simulink model "Microgrid_transition_model_FORFIG"  (R2020a)
settings: Solver=VariableStepAuto  StartTime=0.0  StopTime=16  MaxStep=1e-4  RelTol=1e-3
PreLoadFcn:
  | %run('FC_microgrid_param.m')
  | %load('gen_grid_init.mat')
InitFcn:
  | %load myisoModel_init;
  | run('FC_microgrid_param.m')
  | tic
  | run('CARTinitFcn.m')
  | %caseNo = 2;
  | 
  | %if (caseNo == 1)
  | %set_param(['Isolated_grid_paper_model_022521/SignalGen'], 'ActiveScenario', 'PStep222kW');
  | %else
  | %set_param(['Isolated_grid_paper_model_022521/SignalGen'], 'ActiveScenario', 'QStep222kVAr');
  | 
  | %end;
StopFcn:
  | toc
undefined symbols (not defined in the file): breakpoints1, breakpoints2, cp_table_data, ctrl, D1, Delta, DiscIntNeverNeededParam, DT, FC_BESS, find_system, gcbh, libFC_BESS, LowerLimit, magnitude, oversize, pq_ts, sps_rtmsupport, timer, ts, Ts, Ts_APC, Ts_Control, Ts_Power, UpperLimit
libraries: powerlib x141, powerlib_meascontrol x104, simulink x73, powerlib_extras x60, simulink_extras x16, eePowerMeasurement x9, pi_ctrl x8, sps_avr x7, spsDieselMotorModel x3, SignalEditorBlockLib x2, libLgBattery x1, libFC_PV x1
(part 11 of 14)

== system Microgrid_transition_model_FORFIG/FC_BESS/SMAInverter/85_SMAControl/InvControl/CB_Meas2 ==
  Bus Creator : BusCreator  Inputs=9
  Bus Selector1 : BusSelector  OutputSignals=vabc_line,iabc
  Bus Selector2 : BusSelector  OutputSignals=vabc_line
  Bus Selector3 : BusSelector  OutputSignals=ejwt
  Bus Selector4 : BusSelector  OutputSignals=iabc
  Bus Selector5 : BusSelector  OutputSignals=ejwt
  Bus Selector6 : BusSelector  OutputSignals=vabc_inv
  Bus Selector7 : BusSelector  OutputSignals=ejwt
  Filter : Subsystem
  Filter1 : Subsystem
  InvMeas : Scope  NumInputPorts=7
  Math Function : Math  Operator=square  SignedPower=on  SaturateOnIntegerOverflow=on
  Math Function1 : Math  Operator=square  SignedPower=on  SaturateOnIntegerOverflow=on
  PQ_Calculator : Subsystem
  Sqrt : Sqrt  SaturateOnIntegerOverflow=on
  Sqrt1 : Sqrt  SaturateOnIntegerOverflow=on
  Sum of Elements : Sum  Inputs=+
  Sum of Elements1 : Sum  Inputs=+
  Unit Delay : UnitDelay  SampleTime=-1  HasFrameUpgradeWarning=on
  Unit Delay1 : UnitDelay  SampleTime=-1  HasFrameUpgradeWarning=on
  Unit Delay2 : UnitDelay  SampleTime=-1  HasFrameUpgradeWarning=on
  abc_to_dq0 Transformation : powerlib_extras/Measurements/abc_to_dq0 Transformation
      settings: SourceProductBaseCode=PS
  abc_to_dq0 Transformation1 : powerlib_extras/Measurements/abc_to_dq0 Transformation
      settings: SourceProductBaseCode=PS
  abc_to_dq0 Transformation2 : powerlib_extras/Measurements/abc_to_dq0 Transformation
      settings: SourceProductBaseCode=PS
  tag scope: cb_meas=scoped
  wires:
  PQ_Calculator/2(Q - kVAR) -> Bus Creator/2, InvMeas/6  "q"
  Filter/1(Out1) -> Bus Creator/4, InvMeas/2, Math Function/1
  Filter1/1(Out1) -> Bus Creator/7, InvMeas/4, Math Function1/1
  abc_to_dq0 Transformation1/1 -> Bus Creator/6, InvMeas/3, Filter1/1(In1)  "idq0"
  abc_to_dq0 Transformation/1 -> Bus Creator/3, InvMeas/1, Filter/1(In1)  "vdq0"
  PQ_Calculator/1(P - kW) -> InvMeas/5, Bus Creator/1  "p"
  Unit Delay1/1 -> abc_to_dq0 Transformation1/2
  Unit Delay/1 -> abc_to_dq0 Transformation/2
  [cb_pu] -> Bus Selector4/1
  Sqrt1/1 -> Bus Creator/8  "irms"
  Sum of Elements1/1 -> Sqrt1/1
  Math Function1/1 -> Sum of Elements1/1
  Bus Selector5/1 -> Unit Delay1/1  "<ejwt>"
  [pll] -> Bus Selector5/1
  Bus Selector4/1 -> abc_to_dq0 Transformation1/1  "<iabc>"
  [cb_pu] -> Bus Selector2/1
  Sqrt/1 -> Bus Creator/5  "vrms"
  Sum of Elements/1 -> Sqrt/1
  Math Function/1 -> Sum of Elements/1
  Bus Selector3/1 -> Unit Delay/1  "<ejwt>"
  [pll] -> Bus Selector3/1
  Bus Selector2/1 -> abc_to_dq0 Transformation/1  "<vabc_line>"
  Bus Selector1/2 -> PQ_Calculator/2(Iabc)  "<iabc>"
  Bus Creator/1 -> [cb_meas]
  Bus Selector1/1 -> PQ_Calculator/1(Vabc)  "<vabc_line>"
  [cb_pu] -> Bus Selector1/1
  Bus Selector7/1 -> Unit Delay2/1  "<ejwt>"
  [pll] -> Bus Selector7/1
  [cb_pu] -> Bus Selector6/1
  Bus Selector6/1 -> abc_to_dq0 Transformation2/1  "<vabc_inv>"
  Unit Delay2/1 -> abc_to_dq0 Transformation2/2
  abc_to_dq0 Transformation2/1 -> InvMeas/7, Bus Creator/9  "vdq0_inv"

== system Microgrid_transition_model_FORFIG/FC_BESS/SMAInverter/85_SMAControl/InvControl/CB_pu ==
  Bus Creator : BusCreator  Inputs=3
  Bus Selector1 : BusSelector  OutputSignals=Uabc,Uabc_inv
  Bus Selector2 : BusSelector  OutputSignals=Iabc
  Gain : Gain  Gain=1/Unom/sqrt(2)
  Gain1 : Gain  Gain=1/Inom/sqrt(2)
  Gain2 : Gain  Gain=1/Unom/sqrt(2)
  tag scope: cb_pu=scoped
  wires:
  Gain1/1 -> Bus Creator/3  "iabc"
  Bus Selector2/1 -> Gain1/1  "<Iabc>"
  [inputs] -> Bus Selector2/1
  [inputs] -> Bus Selector1/1
  Bus Selector1/1 -> Gain/1  "<Uabc>"
  Gain/1 -> Bus Creator/1  "vabc_line"
  Bus Creator/1 -> [cb_pu]
  Bus Selector1/2 -> Gain2/1  "<Uabc_inv>"
  Gain2/1 -> Bus Creator/2  "vabc_inv"

== system Microgrid_transition_model_FORFIG/FC_BESS/SMAInverter/85_SMAControl/InvControl/CS_controller ==
  Bias : Bias  Bias=(1.5*Ts)*60*2*pi
  Bus Creator : BusCreator  Inputs=3
  Bus Selector10 : BusSelector  OutputSignals=cb_status,Control_Word.GF_mode
  Bus Selector2 : BusSelector  OutputSignals=udq
  Bus Selector3 : BusSelector  OutputSignals=udq
  Bus Selector5 : BusSelector  OutputSignals=wt
  Constant : Constant  Value=0
  Constant2 : Constant  Value=1.3
  Gain1 : Gain  Gain=-1
  Gain2 : Gain  Gain=Unom*sqrt(2)
  Logical Operator : Logic  AllPortsSameDT=off  OutDataTypeStr=boolean
  Logical Operator1 : Logic  Operator=NOT  AllPortsSameDT=off  OutDataTypeStr=boolean
  Mux1 : Mux  Inputs=2
  Mux3 : Mux  Inputs=2
  Saturation Dynamic : simulink/Discontinuities/Saturation Dynamic  OutMin=[]  OutMax=[]  OutDataTypeStr=Inherit: Same as second input  OutDataType=fixdt(1, 16)  OutScaling=2^-10  DoSatur=off
  Scope : Scope  NumInputPorts=2
  Switch : Switch  Criteria=u2 > Threshold
  Trigonometric Function2 : Trigonometry
  Trigonometric Function3 : Trigonometry  Operator=cos
  dq0_to_abc Transformation : powerlib_extras/Measurements/dq0_to_abc Transformation
      settings: SourceProductBaseCode=PS
  tag scope: inverter=scoped
  wires:
  [use_csi] -> Bus Creator/2  "use_csi"
  Bus Selector3/1 -> Switch/1  "<udq>"
  [I_Ctrl] -> Bus Selector3/1
  Logical Operator/1 -> Switch/2, Scope/1, [use_csi]
  [V_Ctrl] -> Bus Selector2/1
  Bus Selector2/1 -> Switch/3  "<udq>"
  [inputs] -> Bus Selector10/1
  Bus Selector10/2 -> Logical Operator1/1  "<GF_mode>"
  Logical Operator1/1 -> Logical Operator/2
  Bus Selector10/1 -> Logical Operator/1  "<cb_status>"
  Switch/1 -> Mux1/1, Bus Creator/3, Scope/2  "vdq"
  Mux1/1 -> dq0_to_abc Transformation/1
  Constant/1 -> Mux1/2
  Mux3/1 -> [ejwt]
  Trigonometric Function2/1 -> Mux3/1
  Trigonometric Function3/1 -> Mux3/2
  Bias/1 -> Trigonometric Function3/1, Trigonometric Function2/1
  Gain2/1 -> Bus Creator/1  "Uabc_ref"
  Constant2/1 -> Saturation Dynamic/1, Gain1/1
  Gain1/1 -> Saturation Dynamic/3
  Bus Creator/1 -> [inverter]
  dq0_to_abc Transformation/1 -> Saturation Dynamic/2
  [ejwt] -> dq0_to_abc Transformation/2
  Saturation Dynamic/1 -> Gain2/1  "uabc_ref"
  [pll] -> Bus Selector5/1
  Bus Selector5/1 -> Bias/1  "<wt>"

== system Microgrid_transition_model_FORFIG/FC_BESS/SMAInverter/85_SMAControl/InvControl/Droop ==
  Bus Selector1 : BusSelector  OutputSignals=vrms
  Bus Selector2 : BusSelector  OutputSignals=freq
  Bus Selector3 : BusSelector  OutputSignals=p,q,idq0
  Bus Selector9 : BusSelector  OutputSignals=fref,vref,pref,qref  OutputAsBus=on
  Constant : Constant  Value=[0 0]
  Demux : Demux
  Demux1 : Demux
  Droop : Subsystem
  ExtractCoefs : Subsystem
  Gain : Gain  Gain=[1 -1]
  Mux : Mux  Inputs=3
  Mux1 : Mux  Inputs=2
  Mux2 : Mux  Inputs=2
  Scope : Scope  NumInputPorts=4
  Scope1 : Scope  NumInputPorts=4
  Selector1 : Selector  InputPortWidth=4  IndexOptions=Index vector (dialog)  Indices=[1 2]  OutputSizes=1
  Selector2 : Selector  InputPortWidth=3  IndexOptions=Index vector (dialog)  Indices=[1 2]  OutputSizes=1
  Sum1 : Sum  Inputs=-+|
  Sum2 : Sum  Inputs=++|
  Terminator : Terminator
  tag scope: droop=scoped
  wires:
  Demux1/4 -> Scope1/4
  Demux1/1 -> Scope1/1
  Demux1/2 -> Scope1/2
  Demux1/3 -> Scope1/3
  Sum2/1 -> [droop], Demux1/1  "fvpq_meas"
  Gain/1 -> Mux/3
  Selector2/1 -> Gain/1
  Mux2/1 -> Terminator/1
  Bus Selector3/3 -> Selector2/1  "<idq0>"
  Bus Selector3/2 -> Mux2/2  "<q>"
  Bus Selector3/1 -> Mux2/1  "<p>"
  [cb_meas] -> Bus Selector3/1
  Demux/4 -> Scope/4
  Demux/3 -> Scope/3
  Demux/2 -> Scope/2
  Demux/1 -> Scope/1
  Bus Selector2/1 -> Mux/1  "<freq>"
  Bus Selector1/1 -> Mux/2  "<vrms>"
  [pll] -> Bus Selector2/1
  ExtractCoefs/1(Out1) -> Droop/2(droop)
  [inputs] -> ExtractCoefs/1(In1)
  Mux/1 -> Demux/1, Sum1/1  "fvpq_meas"
  [cb_meas] -> Bus Selector1/1
  Bus Selector9/1 -> Selector1/1, Sum2/2
  [inputs] -> Bus Selector9/1
  Droop/1(dFvpq_out) -> Sum2/1
  Sum1/1 -> Droop/1(dfvpq)
  Selector1/1 -> Mux1/1
  Mux1/1 -> Sum1/2
  Constant/1 -> Mux1/2

== system Microgrid_transition_model_FORFIG/FC_BESS/SMAInverter/85_SMAControl/InvControl/PLL ==
  note: Rising and falling edge debounce
  Aligned : simulink/Logic and Bit Operations/Interval Test  IntervalClosedRight=on  uplimit=0.05  IntervalClosedLeft=on  lowlimit=-0.05  OutDataTypeStr=boolean
  Aligned1 : simulink/Logic and Bit Operations/Interval Test  IntervalClosedRight=on  uplimit=1.25  IntervalClosedLeft=on  lowlimit=0.05  OutDataTypeStr=boolean
  Bus Creator : BusCreator  Inputs=5
  Bus Selector10 : BusSelector  OutputSignals=Control_Word.GF_mode
  Bus Selector2 : BusSelector  OutputSignals=vabc_line
  Bus Selector8 : BusSelector  OutputSignals=cb_status
  Constant : Constant  Value=0
  Data Type Conversion : DataTypeConversion
  DebounceAlternative : Subsystem  mask{Tdb_off=0.05, Tdb_on=0.2, Tdb_sample=Ts}
      mask prompts: Tdb_off "Debounce Time When OFF"; Tdb_on "Debounce Time When On"; Tdb_sample "Sample Time"
      mask Display: disp(['Debouncing unit\nTdb when off is ' num2str(Tdb_off) '\nTdb when on is ' num2str(Tdb_on)]);
  Display : Display
  Gain : Gain  Gain=1/60
  Gain1 : Gain  Gain=2*pi*60  SaturateOnIntegerOverflow=on  OutDataTypeStr=Inherit: Same as input  ParamDataTypeStr=Inherit: Same as input
  Logical Operator1 : Logic  AllPortsSameDT=off  OutDataTypeStr=boolean
  Logical Operator2 : Logic  AllPortsSameDT=off  OutDataTypeStr=boolean
  Logical Operator3 : Logic  AllPortsSameDT=off  OutDataTypeStr=boolean
  Logical Operator{4..6,8} (4 alike) : Logic  Operator=NOT  AllPortsSameDT=off  OutDataTypeStr=boolean
  Logical Operator7 : Logic  Operator=OR  AllPortsSameDT=off  OutDataTypeStr=boolean
  Mux3 : Mux  Inputs=2
  PLL (3ph)1 : Subsystem  DialogController=POWERSYS.PowerSysDialog  LoadFcn=sps_rtmsupport('LoadFcn', gcbh);  StartFcn=sps_rtmsupport('StartFcn', gcbh);  StopFcn=sps_rtmsupport('StopFcn', gcbh);  mask(PLL (3ph)){Flim=[55 66], Par_Init=[90, 60], ParK=[pll_kp, pll_ki, 1], TcD=Ts, MaxRateChangeFreq=12, FilterCutOffFreq=25, Ts=Ts, AGC=off}
      mask prompts: Flim "Minimum frequency (Hz):"; Par_Init "Initial inputs [ Phase (degrees), Frequency (Hz) ]:"; ParK "Regulator gains [ Kp, Ki, Kd ]:"; TcD "Time constant for derivative action (s):"; MaxRateChangeFreq "Maximum rate of change of frequency (Hz/s):"; FilterCutOffFreq "Filter cut-off frequency for frequency measurement (Hz):"; Ts "Sample time:"; AGC "Enable automatic gain control"
      mask help:
      | This Phase Locked Loop (PLL) system can be used  to synchronize on a set of variable frequency, three-phase sinusoidal signals. If the Automatic Gain Control is enabled, the input (phase error) of the PLL regulator is scaled according to the input signals magnitude.
      |
      | For optimal performance, set regulator gains [ Kp Ki  Kd ] = [ 180  3200  1 ] and check the Enable Automatic Gain Control parameter.
      |
      | Input : Vector containing the normalized three-phase signals [Va Vb Vc]
      | Output 1:  Measured frequency (Hz) = w/(2pi)
      | Output 2:  Ramp w.t varying between  0 and 2*pi, synchronized on zero crossings of the fundamental (positive-sequence) of phase A.
      mask init:
      | %block=gcb;
      | %[WantBlockChoice,Ts,sps] = powericon('PLL3phInit',block,Fmin,Par_Init,ParK,TcD, MaxRateChangeFreq, FilterCutOffFreq, AGC,Ts);
      | %powericon('SetInternalModels','set',block,WantBlockChoice);
      settings: CopyFcn=sps_rtmsupport('CopyFcn', gcbh);  DeleteFcn=sps_rtmsupport('DeleteFcn', gcbh);  UndoDeleteFcn=sps_rtmsupport('UndoDeleteFcn', gcbh);  ModelCloseFcn=sps_rtmsupport('ModelCloseFcn', gcbh);  PreSaveFcn=sps_rtmsupport('PreSaveFcn', gcbh);  PostSaveFcn=sps_rtmsupport('PostSaveFcn', gcbh);  NameChangeFcn=sps_rtmsupport('NameChangeFcn', gcbh);  PreCopyFcn=sps_rtmsupport('PreCopyFcn', gcbh);  CloseFcn=sps_rtmsupport('CloseFcn', gcbh);  PreDeleteFcn=sps_rtmsupport('PreDeleteFcn', gcbh);
      settings: OpenFcn=|
      | power_openblockproxy();
      | sps_rtmsupport('OpenFcn', gcbh, [8]);
      mask Help: helpview(psbhelp);
  Scope : Scope  NumInputPorts=5
  Selector1 : Selector  InputPortWidth=3  IndexOptions=Index vector (dialog)  Indices=1  OutputSizes=1
  Selector2 : Selector  InputPortWidth=3  IndexOptions=Index vector (dialog)  Indices=2  OutputSizes=1
  Selector3 : Selector  InputPortWidth=4  IndexOptions=Index vector (dialog)  Indices=[1]  OutputSizes=1
  Switch : Switch  Criteria=u2 > Threshold
  Terminator : Terminator
  Trigonometric Function2 : Trigonometry
  Trigonometric Function3 : Trigonometry  Operator=cos
  VCO : Subsystem
  tag scope: pll=scoped
  wires:
  Switch/1 -> Bus Creator/3, Scope/5, Trigonometric Function2/1, Trigonometric Function3/1  "wt"
  PLL (3ph)1/3(dq0) -> Selector2/1, Selector1/1
  Logical Operator7/1 -> Scope/1, [use_pll]  "use_pll"
  Logical Operator3/1 -> Logical Operator7/2
  Logical Operator5/1 -> Logical Operator3/2
  Logical Operator4/1 -> Logical Operator3/1
  Bus Selector10/1 -> Logical Operator5/1  "<GF_mode>"
  Logical Operator1/1 -> Logical Operator7/1
  [lock] -> Logical Operator1/2
  [cb_open] -> Logical Operator1/1, Scope/4, Logical Operator4/1  "cb_open"
  Bus Selector8/1 -> Logical Operator8/1  "<cb_status>"
  Logical Operator8/1 -> Display/1, [cb_open]
  [inputs] -> Bus Selector8/1
  [inputs] -> Bus Selector10/1
  Trigonometric Function3/1 -> Mux3/2
  Trigonometric Function2/1 -> Mux3/1
  Mux3/1 -> Bus Creator/4  "ejwt"
  Logical Operator6/1 -> Switch/2
  [use_pll] -> VCO/2(rst), Logical Operator6/1
  VCO/1(theta) -> Switch/1
  Gain1/1 -> VCO/1(w)
  [ref_lim] -> Selector3/1
  Selector3/1 -> Scope/3, Gain1/1
  Gain/1 -> Bus Creator/1  "freq"
  PLL (3ph)1/2(wt) -> VCO/3(init), Switch/3  "wt"
  Bus Selector2/1 -> PLL (3ph)1/1(abc)  "<vabc_line>"
  [cb_pu] -> Bus Selector2/1
  Data Type Conversion/1 -> DebounceAlternative/1(In)
  Constant/1 -> DebounceAlternative/2(Rst)
  DebounceAlternative/2(IntOut) -> Terminator/1
  Logical Operator2/1 -> Data Type Conversion/1
  Selector2/1 -> Aligned/1
  Selector1/1 -> Aligned1/1
  Aligned1/1 -> Logical Operator2/2
  Aligned/1 -> Logical Operator2/1
  DebounceAlternative/1(Out) -> Scope/2, [lock], Bus Creator/5  "lock"
  PLL (3ph)1/1(Freq) -> Gain/1, Bus Creator/2  "Freq"
  Bus Creator/1 -> [pll]

== system Microgrid_transition_model_FORFIG/FC_BESS/SMAInverter/85_SMAControl/InvControl/Ref_Limiting ==
  Constant : Constant
  Constant1 : Constant  Value=-1
  Demux : Demux
  RefLimiting : Subsystem
  Scope : Scope  NumInputPorts=4
  tag scope: ref_lim=scoped
  wires:
  Demux/4 -> Scope/4
  Demux/3 -> Scope/3
  Demux/2 -> Scope/2
  Demux/1 -> Scope/1
  [droop] -> RefLimiting/1(fvpq_in)
  Constant/1 -> RefLimiting/2(p_max)
  Constant1/1 -> RefLimiting/3(p_min)
  RefLimiting/1(fvpq_out) -> Demux/1, [ref_lim]  "FVPQ"

== system Microgrid_transition_model_FORFIG/MODEL STABILIZER/AllStringInverters/Stab_control/InvControl/40_V_Control ==
  Add1 : Sum  Inputs=+-
  Bus Creator : BusCreator  Inputs=1
  Bus Selector1 : BusSelector  OutputSignals=vdq0_inv  OutputAsBus=on
  Bus Selector8 : BusSelector  OutputSignals=use_csi,vdq
  Constant1 : Constant  Value=double(0)
  Constant2 : Constant  Value=10  OutDataTypeStr=double
  Demux : Demux  Outputs=2
  Demux1 : Demux  Outputs=2
  Logical Operator : Logic  Operator=NOT  Inputs=1  AllPortsSameDT=off  OutDataTypeStr=boolean
  Manual Switch2 : ManualSwitch  CurrentSetting=0
  Mux2 : Mux  Inputs=2
  Mux8 : Mux  Inputs=2
  PI_controller_with_reset : pi_ctrl/PI_controller_with_reset  Kp=0.0005  Ti=0.02  Ts=Ts  Iup=1.5  Idown=0  PIup=1.5  PIdown=0
  PI_controller_with_reset1 : pi_ctrl/PI_controller_with_reset  Kp=0.0005  Ti=0.02  Ts=Ts  Iup=1.5  Idown=-1  PIup=1.5  PIdown=-1
  Scope : Scope  NumInputPorts=4
  Selector : Selector  InputPortWidth=4  IndexOptions=Index vector (dialog)  Indices=2  OutputSizes=1
  Selector2 : Selector  InputPortWidth=3  IndexOptions=Index vector (dialog)  Indices=[1 2]  OutputSizes=1
  Subsystem : Subsystem  mask{Ts=Ts}
      mask prompts: Ts "Sampling time"
  Unit Delay : UnitDelay  SampleTime=-1  HasFrameUpgradeWarning=on
  Unit Delay1 : UnitDelay  InitialCondition=[0 0]  SampleTime=-1  HasFrameUpgradeWarning=on
  tag scope: V_Ctrl=scoped
  wires:
  [ref_lim] -> Selector/1
  Bus Creator/1 -> [V_Ctrl]
  Mux8/1 -> Scope/3, Unit Delay/1, Bus Creator/1  "udq"
  [cb_meas] -> Bus Selector1/1
  Bus Selector1/1 -> Selector2/1
  PI_controller_with_reset/1 -> Mux8/1, Scope/4
  Demux1/1 -> PI_controller_with_reset/1
  Demux1/2 -> PI_controller_with_reset1/1
  Add1/1 -> Demux1/1
  Subsystem/1(out) -> Add1/1, Scope/1
  Manual Switch2/1 -> Add1/2, Scope/2
  Selector/1 -> Mux2/1
  Constant1/1 -> Mux2/2
  [inverter] -> Bus Selector8/1
  PI_controller_with_reset1/1 -> Mux8/2
  Logical Operator/1 -> PI_controller_with_reset1/2, PI_controller_with_reset/2
  Bus Selector8/2 -> Unit Delay1/1  "<vdq>"
  Demux/1 -> PI_controller_with_reset/3
  Demux/2 -> PI_controller_with_reset1/3
  Selector2/1 -> Manual Switch2/2
  Unit Delay/1 -> Manual Switch2/1
  Bus Selector8/1 -> Subsystem/2(rst), Logical Operator/1  "<use_csi>"
  Mux2/1 -> Subsystem/1(in)
  Constant2/1 -> Subsystem/4(rate)
  Unit Delay1/1 -> Subsystem/3(init), Demux/1

== system Microgrid_transition_model_FORFIG/MODEL STABILIZER/AllStringInverters/Stab_control/InvControl/50_I_Control ==
  Add1 : Sum  Inputs=+-
  Bus Creator : BusCreator  Inputs=1
  Bus Selector1 : BusSelector  OutputSignals=idq0  OutputAsBus=on
  Bus Selector2 : BusSelector  OutputSignals=use_csi,vdq
  Bus Selector3 : BusSelector  OutputSignals=vdq0_inv  OutputAsBus=on
  Constant : Constant  Value=10  OutDataTypeStr=double
  Demux : Demux  Outputs=2
  Demux1 : Demux  Outputs=2
  Filter : Subsystem
  Filter1 : Subsystem
  Gain : Gain
  Gain1 : Gain
  Logical Operator : Logic  Operator=NOT  Inputs=1  AllPortsSameDT=off  OutDataTypeStr=boolean
  Mux8 : Mux  Inputs=2
  PI_controller_with_reset : pi_ctrl/PI_controller_with_reset  Kp=cc_kp  Ti=cc_Ti  Ts=Ts  Iup=1.5  Idown=-0.5  PIup=1.5  PIdown=-0.5
  PI_controller_with_reset1 : pi_ctrl/PI_controller_with_reset  Kp=cc_kp  Ti=0.6e-3*100  Ts=Ts  Iup=1  Idown=-1  PIup=1  PIdown=-1
  Scope : Scope  NumInputPorts=3
  Selector : Selector  InputPortWidth=4  IndexOptions=Index vector (dialog)  Indices=[3 4]  OutputSizes=1
  Selector1 : Selector  InputPortWidth=3  IndexOptions=Index vector (dialog)  Indices=[1 2]  OutputSizes=1
  Selector2 : Selector  InputPortWidth=3  IndexOptions=Index vector (dialog)  Indices=[1 2]  OutputSizes=1
  Subsystem : Subsystem  mask{Ts=Ts}
      mask prompts: Ts "Sampling time"
  Sum : Sum  Inputs=|++
  Sum1 : Sum  Inputs=|+-
  Unit Delay : UnitDelay  SampleTime=-1  HasFrameUpgradeWarning=on
  tag scope: I_Ctrl=scoped
  wires:
  Gain1/1 -> Sum/2
  Gain/1 -> Sum1/2
  Filter1/1(Out1) -> Gain/1, Gain1/1
  Selector1/1 -> Filter1/1(In1)
  Bus Selector3/1 -> Selector1/1
  [cb_meas] -> Bus Selector3/1
  Sum1/1 -> Demux/1  "udq"
  Mux8/1 -> Scope/2, Sum/1  "udq"
  Filter/1(Out1) -> Add1/2
  Selector2/1 -> Filter/1(In1), Subsystem/3(init)
  Subsystem/1(out) -> Add1/1
  Add1/1 -> Demux1/1
  Demux1/2 -> PI_controller_with_reset1/1
  Demux1/1 -> PI_controller_with_reset/1
  PI_controller_with_reset/1 -> Mux8/1
  Bus Selector1/1 -> Selector2/1
  [cb_meas] -> Bus Selector1/1
  Sum/1 -> Bus Creator/1, Scope/3  "udq"
  Bus Creator/1 -> [I_Ctrl]
  [ref_lim] -> Selector/1
  [inverter] -> Bus Selector2/1
  Bus Selector2/1 -> PI_controller_with_reset/2, Scope/1, PI_controller_with_reset1/2, Logical Operator/1  "<use_csi>"
  Bus Selector2/2 -> Unit Delay/1  "<vdq>"
  Demux/1 -> PI_controller_with_reset/3
  Demux/2 -> PI_controller_with_reset1/3
  Selector/1 -> Subsystem/1(in)
  Constant/1 -> Subsystem/4(rate)
  Logical Operator/1 -> Subsystem/2(rst)
  Unit Delay/1 -> Sum1/1
  PI_controller_with_reset1/1 -> Mux8/2

== system Microgrid_transition_model_FORFIG/MODEL STABILIZER/AllStringInverters/Stab_control/InvControl/CB_Meas2 ==
  Bus Creator : BusCreator  Inputs=9
  Bus Selector1 : BusSelector  OutputSignals=vabc_line,iabc
  Bus Selector2 : BusSelector  OutputSignals=vabc_line
  Bus Selector3 : BusSelector  OutputSignals=ejwt
  Bus Selector4 : BusSelector  OutputSignals=iabc
  Bus Selector5 : BusSelector  OutputSignals=ejwt
  Bus Selector6 : BusSelector  OutputSignals=vabc_inv
  Bus Selector7 : BusSelector  OutputSignals=ejwt
  Filter : Subsystem
  Filter1 : Subsystem
  Math Function : Math  Operator=square  SignedPower=on  SaturateOnIntegerOverflow=on
  Math Function1 : Math  Operator=square  SignedPower=on  SaturateOnIntegerOverflow=on
  PQ_Calculator : Subsystem
  Sqrt : Sqrt  SaturateOnIntegerOverflow=on
  Sqrt1 : Sqrt  SaturateOnIntegerOverflow=on
  Sum of Elements : Sum  Inputs=+
  Sum of Elements1 : Sum  Inputs=+
  Unit Delay : UnitDelay  SampleTime=-1  HasFrameUpgradeWarning=on
  Unit Delay1 : UnitDelay  SampleTime=-1  HasFrameUpgradeWarning=on
  Unit Delay2 : UnitDelay  SampleTime=-1  HasFrameUpgradeWarning=on
  abc_to_dq0 Transformation : powerlib_extras/Measurements/abc_to_dq0 Transformation
      settings: SourceProductBaseCode=PS
  abc_to_dq0 Transformation1 : powerlib_extras/Measurements/abc_to_dq0 Transformation
      settings: SourceProductBaseCode=PS
  abc_to_dq0 Transformation2 : powerlib_extras/Measurements/abc_to_dq0 Transformation
      settings: SourceProductBaseCode=PS
  tag scope: cb_meas=scoped
  wires:
  abc_to_dq0 Transformation2/1 -> Bus Creator/9  "vdq0_inv"
  Unit Delay2/1 -> abc_to_dq0 Transformation2/2
  Bus Selector6/1 -> abc_to_dq0 Transformation2/1  "<vabc_inv>"
  [cb_pu] -> Bus Selector6/1
  [pll] -> Bus Selector7/1
  Bus Selector7/1 -> Unit Delay2/1  "<ejwt>"
  [cb_pu] -> Bus Selector1/1
  Bus Selector1/1 -> PQ_Calculator/1(Vabc)  "<vabc_line>"
  Bus Creator/1 -> [cb_meas]
  Bus Selector1/2 -> PQ_Calculator/2(Iabc)  "<iabc>"
  Bus Selector2/1 -> abc_to_dq0 Transformation/1  "<vabc_line>"
  [pll] -> Bus Selector3/1
  Bus Selector3/1 -> Unit Delay/1  "<ejwt>"
  Math Function/1 -> Sum of Elements/1
  Sum of Elements/1 -> Sqrt/1
  Sqrt/1 -> Bus Creator/5  "vrms"
  [cb_pu] -> Bus Selector2/1
  Bus Selector4/1 -> abc_to_dq0 Transformation1/1  "<iabc>"
  [pll] -> Bus Selector5/1
  Bus Selector5/1 -> Unit Delay1/1  "<ejwt>"
  Math Function1/1 -> Sum of Elements1/1
  Sum of Elements1/1 -> Sqrt1/1
  Sqrt1/1 -> Bus Creator/8  "irms"
  [cb_pu] -> Bus Selector4/1
  Unit Delay/1 -> abc_to_dq0 Transformation/2
  Unit Delay1/1 -> abc_to_dq0 Transformation1/2
  PQ_Calculator/1(P - kW) -> Bus Creator/1  "p"
  abc_to_dq0 Transformation/1 -> Filter/1(In1), Bus Creator/3  "vdq0"
  abc_to_dq0 Transformation1/1 -> Filter1/1(In1), Bus Creator/6  "idq0"
  Filter1/1(Out1) -> Math Function1/1, Bus Creator/7
  Filter/1(Out1) -> Math Function/1, Bus Creator/4
  PQ_Calculator/2(Q - kVAR) -> Bus Creator/2  "q"

== system Microgrid_transition_model_FORFIG/MODEL STABILIZER/AllStringInverters/Stab_control/InvControl/CB_pu ==
  Bus Creator : BusCreator  Inputs=3
  Bus Selector1 : BusSelector  OutputSignals=Uabc,Uabc_inv
  Bus Selector2 : BusSelector  OutputSignals=Iabc
  Gain : Gain  Gain=1/Unom/sqrt(2)
  Gain1 : Gain  Gain=1/Inom/sqrt(2)
  Gain2 : Gain  Gain=1/Unom/sqrt(2)
  tag scope: cb_pu=scoped
  wires:
  Gain2/1 -> Bus Creator/2  "vabc_inv"
  Bus Selector1/2 -> Gain2/1  "<Uabc_inv>"
  Bus Creator/1 -> [cb_pu]
  Gain/1 -> Bus Creator/1  "vabc_line"
  Bus Selector1/1 -> Gain/1  "<Uabc>"
  [inputs] -> Bus Selector1/1
  [inputs] -> Bus Selector2/1
  Bus Selector2/1 -> Gain1/1  "<Iabc>"
  Gain1/1 -> Bus Creator/3  "iabc"

== system Microgrid_transition_model_FORFIG/MODEL STABILIZER/AllStringInverters/Stab_control/InvControl/CS_controller ==
  Bias : Bias  Bias=(1.5*Ts)*60*2*pi
  Bus Creator : BusCreator  Inputs=3
  Bus Selector10 : BusSelector  OutputSignals=cb_status,Control_Word.GF_mode
  Bus Selector2 : BusSelector  OutputSignals=udq
  Bus Selector3 : BusSelector  OutputSignals=udq
  Bus Selector5 : BusSelector  OutputSignals=wt
  Constant : Constant  Value=0
  Constant2 : Constant  Value=1.3
  Gain1 : Gain  Gain=-1
  Gain2 : Gain  Gain=Unom*sqrt(2)
  Logical Operator : Logic  AllPortsSameDT=off  OutDataTypeStr=boolean
  Logical Operator1 : Logic  Operator=NOT  AllPortsSameDT=off  OutDataTypeStr=boolean
  Mux1 : Mux  Inputs=2
  Mux3 : Mux  Inputs=2
  Saturation Dynamic : simulink/Discontinuities/Saturation Dynamic  OutMin=[]  OutMax=[]  OutDataTypeStr=Inherit: Same as second input  OutDataType=fixdt(1, 16)  OutScaling=2^-10  DoSatur=off
  Scope : Scope  NumInputPorts=2
  Switch : Switch  Criteria=u2 > Threshold
  Trigonometric Function2 : Trigonometry
  Trigonometric Function3 : Trigonometry  Operator=cos
  dq0_to_abc Transformation : powerlib_extras/Measurements/dq0_to_abc Transformation
      settings: SourceProductBaseCode=PS
  tag scope: inverter=scoped
  wires:
  Bus Selector5/1 -> Bias/1  "<wt>"
  [pll] -> Bus Selector5/1
  Saturation Dynamic/1 -> Gain2/1  "uabc_ref"
  [ejwt] -> dq0_to_abc Transformation/2
  dq0_to_abc Transformation/1 -> Saturation Dynamic/2
  Bus Creator/1 -> [inverter]
  Gain1/1 -> Saturation Dynamic/3
  Constant2/1 -> Gain1/1, Saturation Dynamic/1
  Gain2/1 -> Bus Creator/1  "Uabc_ref"
  Bias/1 -> Trigonometric Function2/1, Trigonometric Function3/1
  Trigonometric Function3/1 -> Mux3/2
  Trigonometric Function2/1 -> Mux3/1
  Mux3/1 -> [ejwt]
  Constant/1 -> Mux1/2
  Mux1/1 -> dq0_to_abc Transformation/1
  Switch/1 -> Scope/2, Bus Creator/3, Mux1/1  "vdq"
  Bus Selector10/1 -> Logical Operator/1  "<cb_status>"
  Logical Operator1/1 -> Logical Operator/2
  Bus Selector10/2 -> Logical Operator1/1  "<GF_mode>"
  [inputs] -> Bus Selector10/1
  Bus Selector2/1 -> Switch/3  "<udq>"
  [V_Ctrl] -> Bus Selector2/1
  Logical Operator/1 -> [use_csi], Scope/1, Switch/2
  [I_Ctrl] -> Bus Selector3/1
  Bus Selector3/1 -> Switch/1  "<udq>"
  [use_csi] -> Bus Creator/2  "use_csi"

== system Microgrid_transition_model_FORFIG/MODEL STABILIZER/AllStringInverters/Stab_control/InvControl/Droop ==
  Bus Selector1 : BusSelector  OutputSignals=vrms
  Bus Selector2 : BusSelector  OutputSignals=freq
  Bus Selector3 : BusSelector  OutputSignals=p,q,idq0
  Bus Selector9 : BusSelector  OutputSignals=fref,vref,pref,qref  OutputAsBus=on
  Constant : Constant  Value=[0 0]
  Demux : Demux
  Demux1 : Demux
  Droop : Subsystem
  ExtractCoefs : Subsystem
  Gain : Gain  Gain=[1 -1]
  Mux : Mux  Inputs=3
  Mux1 : Mux  Inputs=2
  Mux2 : Mux  Inputs=2
  Scope : Scope  NumInputPorts=4
  Scope1 : Scope  NumInputPorts=4
  Selector1 : Selector  InputPortWidth=4  IndexOptions=Index vector (dialog)  Indices=[1 2]  OutputSizes=1
  Selector2 : Selector  InputPortWidth=3  IndexOptions=Index vector (dialog)  Indices=[1 2]  OutputSizes=1
  Sum1 : Sum  Inputs=-+|
  Sum2 : Sum  Inputs=++|
  Terminator : Terminator
  tag scope: droop=scoped
  wires:
  Constant/1 -> Mux1/2
  Mux1/1 -> Sum1/2
  Selector1/1 -> Mux1/1
  Sum1/1 -> Droop/1(dfvpq)
  Droop/1(dFvpq_out) -> Sum2/1
  [inputs] -> Bus Selector9/1
  Bus Selector9/1 -> Sum2/2, Selector1/1
  [cb_meas] -> Bus Selector1/1
  Mux/1 -> Sum1/1, Demux/1  "fvpq_meas"
  [inputs] -> ExtractCoefs/1(In1)
  ExtractCoefs/1(Out1) -> Droop/2(droop)
  [pll] -> Bus Selector2/1
  Bus Selector1/1 -> Mux/2  "<vrms>"
  Bus Selector2/1 -> Mux/1  "<freq>"
  Demux/1 -> Scope/1
  Demux/2 -> Scope/2
  Demux/3 -> Scope/3
  Demux/4 -> Scope/4
  [cb_meas] -> Bus Selector3/1
  Bus Selector3/1 -> Mux2/1  "<p>"
  Bus Selector3/2 -> Mux2/2  "<q>"
  Bus Selector3/3 -> Selector2/1  "<idq0>"
  Mux2/1 -> Terminator/1
  Selector2/1 -> Gain/1
  Gain/1 -> Mux/3
  Sum2/1 -> Demux1/1, [droop]  "fvpq_meas"
  Demux1/3 -> Scope1/3
  Demux1/2 -> Scope1/2
  Demux1/1 -> Scope1/1
  Demux1/4 -> Scope1/4

== system Microgrid_transition_model_FORFIG/MODEL STABILIZER/AllStringInverters/Stab_control/InvControl/PLL ==
  note: Rising and falling edge debounce
  Aligned : simulink/Logic and Bit Operations/Interval Test  IntervalClosedRight=on  uplimit=0.05  IntervalClosedLeft=on  lowlimit=-0.05  OutDataTypeStr=boolean
  Aligned1 : simulink/Logic and Bit Operations/Interval Test  IntervalClosedRight=on  uplimit=1.25  IntervalClosedLeft=on  lowlimit=0.05  OutDataTypeStr=boolean
  Bus Creator : BusCreator  Inputs=5
  Bus Selector10 : BusSelector  OutputSignals=Control_Word.GF_mode
  Bus Selector2 : BusSelector  OutputSignals=vabc_line
  Bus Selector8 : BusSelector  OutputSignals=cb_status
  Constant : Constant  Value=0
  Data Type Conversion : DataTypeConversion
  DebounceAlternative : Subsystem  mask{Tdb_off=0.05, Tdb_on=0.2, Tdb_sample=Ts}
      mask prompts: Tdb_off "Debounce Time When OFF"; Tdb_on "Debounce Time When On"; Tdb_sample "Sample Time"
      mask Display: disp(['Debouncing unit\nTdb when off is ' num2str(Tdb_off) '\nTdb when on is ' num2str(Tdb_on)]);
  Display : Display
  Gain : Gain  Gain=1/60
  Gain1 : Gain  Gain=2*pi*60  SaturateOnIntegerOverflow=on  OutDataTypeStr=Inherit: Same as input  ParamDataTypeStr=Inherit: Same as input
  Logical Operator1 : Logic  AllPortsSameDT=off  OutDataTypeStr=boolean
  Logical Operator2 : Logic  AllPortsSameDT=off  OutDataTypeStr=boolean
  Logical Operator3 : Logic  AllPortsSameDT=off  OutDataTypeStr=boolean
  Logical Operator{4..6,8} (4 alike) : Logic  Operator=NOT  AllPortsSameDT=off  OutDataTypeStr=boolean
  Logical Operator7 : Logic  Operator=OR  AllPortsSameDT=off  OutDataTypeStr=boolean
  Mux3 : Mux  Inputs=2
  PLL (3ph)1 : Subsystem  DialogController=POWERSYS.PowerSysDialog  LoadFcn=sps_rtmsupport('LoadFcn', gcbh);  StartFcn=sps_rtmsupport('StartFcn', gcbh);  StopFcn=sps_rtmsupport('StopFcn', gcbh);  mask(PLL (3ph)){Flim=[55 66], Par_Init=[90, 60], ParK=[pll_kp, pll_ki, 1], TcD=Ts, MaxRateChangeFreq=12, FilterCutOffFreq=25, Ts=Ts, AGC=off}
      mask prompts: Flim "Minimum frequency (Hz):"; Par_Init "Initial inputs [ Phase (degrees), Frequency (Hz) ]:"; ParK "Regulator gains [ Kp, Ki, Kd ]:"; TcD "Time constant for derivative action (s):"; MaxRateChangeFreq "Maximum rate of change of frequency (Hz/s):"; FilterCutOffFreq "Filter cut-off frequency for frequency measurement (Hz):"; Ts "Sample time:"; AGC "Enable automatic gain control"
      mask help:
      | This Phase Locked Loop (PLL) system can be used  to synchronize on a set of variable frequency, three-phase sinusoidal signals. If the Automatic Gain Control is enabled, the input (phase error) of the PLL regulator is scaled according to the input signals magnitude.
      |
      | For optimal performance, set regulator gains [ Kp Ki  Kd ] = [ 180  3200  1 ] and check the Enable Automatic Gain Control parameter.
      |
      | Input : Vector containing the normalized three-phase signals [Va Vb Vc]
      | Output 1:  Measured frequency (Hz) = w/(2pi)
      | Output 2:  Ramp w.t varying between  0 and 2*pi, synchronized on zero crossings of the fundamental (positive-sequence) of phase A.
      mask init:
      | %block=gcb;
      | %[WantBlockChoice,Ts,sps] = powericon('PLL3phInit',block,Fmin,Par_Init,ParK,TcD, MaxRateChangeFreq, FilterCutOffFreq, AGC,Ts);
      | %powericon('SetInternalModels','set',block,WantBlockChoice);
      settings: CopyFcn=sps_rtmsupport('CopyFcn', gcbh);  DeleteFcn=sps_rtmsupport('DeleteFcn', gcbh);  UndoDeleteFcn=sps_rtmsupport('UndoDeleteFcn', gcbh);  ModelCloseFcn=sps_rtmsupport('ModelCloseFcn', gcbh);  PreSaveFcn=sps_rtmsupport('PreSaveFcn', gcbh);  PostSaveFcn=sps_rtmsupport('PostSaveFcn', gcbh);  NameChangeFcn=sps_rtmsupport('NameChangeFcn', gcbh);  PreCopyFcn=sps_rtmsupport('PreCopyFcn', gcbh);  CloseFcn=sps_rtmsupport('CloseFcn', gcbh);  PreDeleteFcn=sps_rtmsupport('PreDeleteFcn', gcbh);
      settings: OpenFcn=|
      | power_openblockproxy();
      | sps_rtmsupport('OpenFcn', gcbh, [8]);
      mask Help: helpview(psbhelp);
  Scope : Scope  NumInputPorts=5
  Selector1 : Selector  InputPortWidth=3  IndexOptions=Index vector (dialog)  Indices=1  OutputSizes=1
  Selector2 : Selector  InputPortWidth=3  IndexOptions=Index vector (dialog)  Indices=2  OutputSizes=1
  Selector3 : Selector  InputPortWidth=4  IndexOptions=Index vector (dialog)  Indices=[1]  OutputSizes=1
  Switch : Switch  Criteria=u2 > Threshold
  Terminator : Terminator
  Trigonometric Function2 : Trigonometry
  Trigonometric Function3 : Trigonometry  Operator=cos
  VCO : Subsystem
  tag scope: pll=scoped
  wires:
  Bus Creator/1 -> [pll]
  PLL (3ph)1/1(Freq) -> Bus Creator/2, Gain/1  "Freq"
  DebounceAlternative/1(Out) -> Bus Creator/5, [lock], Scope/2  "lock"
  Aligned/1 -> Logical Operator2/1
  Aligned1/1 -> Logical Operator2/2
  Selector1/1 -> Aligned1/1
  Selector2/1 -> Aligned/1
  Logical Operator2/1 -> Data Type Conversion/1
  DebounceAlternative/2(IntOut) -> Terminator/1
  Constant/1 -> DebounceAlternative/2(Rst)
  Data Type Conversion/1 -> DebounceAlternative/1(In)
  [cb_pu] -> Bus Selector2/1
  Bus Selector2/1 -> PLL (3ph)1/1(abc)  "<vabc_line>"
  PLL (3ph)1/2(wt) -> Switch/3, VCO/3(init)  "wt"
  Gain/1 -> Bus Creator/1  "freq"
  Selector3/1 -> Gain1/1, Scope/3
  [ref_lim] -> Selector3/1
  Gain1/1 -> VCO/1(w)
  VCO/1(theta) -> Switch/1
  [use_pll] -> Logical Operator6/1, VCO/2(rst)
  Logical Operator6/1 -> Switch/2
  Mux3/1 -> Bus Creator/4  "ejwt"
  Trigonometric Function2/1 -> Mux3/1
  Trigonometric Function3/1 -> Mux3/2
  [inputs] -> Bus Selector10/1
  [inputs] -> Bus Selector8/1
  Logical Operator8/1 -> [cb_open], Display/1
  Bus Selector8/1 -> Logical Operator8/1  "<cb_status>"
  [cb_open] -> Logical Operator4/1, Scope/4, Logical Operator1/1  "cb_open"
  [lock] -> Logical Operator1/2
  Logical Operator1/1 -> Logical Operator7/1
  Bus Selector10/1 -> Logical Operator5/1  "<GF_mode>"
  Logical Operator4/1 -> Logical Operator3/1
  Logical Operator5/1 -> Logical Operator3/2
  Logical Operator3/1 -> Logical Operator7/2
  Logical Operator7/1 -> [use_pll], Scope/1  "use_pll"
  PLL (3ph)1/3(dq0) -> Selector1/1, Selector2/1
  Switch/1 -> Trigonometric Function3/1, Trigonometric Function2/1, Scope/5, Bus Creator/3  "wt"

== system Microgrid_transition_model_FORFIG/MODEL STABILIZER/AllStringInverters/Stab_control/InvControl/Ref_Limiting ==
  Constant : Constant
  Constant1 : Constant  Value=-1
  Demux : Demux
  RefLimiting : Subsystem
  Scope : Scope  NumInputPorts=4
  tag scope: ref_lim=scoped
  wires:
  RefLimiting/1(fvpq_out) -> [ref_lim], Demux/1  "FVPQ"
  Constant1/1 -> RefLimiting/3(p_min)
  Constant/1 -> RefLimiting/2(p_max)
  [droop] -> RefLimiting/1(fvpq_in)
  Demux/1 -> Scope/1
  Demux/2 -> Scope/2
  Demux/3 -> Scope/3
  Demux/4 -> Scope/4

== system Microgrid_transition_model_FORFIG/Wind Turbine Type 4/APC (atomic)1/Inertial Response (to df)/FBIC/S&H1 ==
  In : Inport
  S : Inport  Port=2
  Data Type Conversion : DataTypeConversion  OutDataTypeStr=boolean
  IC=ic : Memory  InitialCondition=ic  InheritSampleTime=on  LinearizeAsDelay=on
  Switch : Switch  Threshold=0.5  SaturateOnIntegerOverflow=on  InputSameDT=on
  Out : Outport  InitialOutput=0
  wires:
  Switch/1 -> IC=ic/1, Out/1
  S/1 -> Data Type Conversion/1
  Data Type Conversion/1 -> Switch/2
  IC=ic/1 -> Switch/3
  In/1 -> Switch/1

== system Microgrid_transition_model_FORFIG/Wind Turbine Type 4/APC (atomic)1/Inertial Response (to df)/Lock2/S&H ==
  In : Inport
  S : Inport  Port=2
  Data Type Conversion : DataTypeConversion  OutDataTypeStr=boolean
  IC=ic : Memory  InitialCondition=ic  InheritSampleTime=on  LinearizeAsDelay=on
  Switch : Switch  Threshold=0.5  SaturateOnIntegerOverflow=on  InputSameDT=on
  Out : Outport  InitialOutput=0
  wires:
  Switch/1 -> IC=ic/1, Out/1
  S/1 -> Data Type Conversion/1
  Data Type Conversion/1 -> Switch/2
  IC=ic/1 -> Switch/3
  In/1 -> Switch/1

== system Microgrid_transition_model_FORFIG/Wind Turbine Type 4/Control/Measurement and Transformation/Discrete 3-phase PLL-Driven Positive-Sequence Active & Reactive Power/Discrete 3-phase PLL-Driven Positive-Sequence Fundamental Value ==
  note: Pierre Giroux, Gilbert Sybille
      | Power System Simulation Laboratory
      | IREQ, Hydro-Quebc
  note: Discrete 3-phase PLL-Driven Positive-Sequence Fundamental Value
  Freq : Inport
  w : Inport  Port=2  PortDimensions=1
  abc : Inport  Port=3  PortDimensions=3
  Cartesian to Polar : simulink_extras/Transformations/Cartesian to Polar
  Demux : Demux  Outputs=3
      settings: DisplayOption=none
  Discrete Variable Frequency Mean value1 : Subsystem  mask(Discrete Variable-Frequency Mean Value){Finit=Finit, Fmin=Fmin, Vinit=Imag_Init, Ts=Ts}
      mask prompts: Finit "Initial frequency (Hz):"; Fmin "Minimum frequency (Hz):"; Vinit "Initial input (DC component):"; Ts "Sample time:"
      mask help:
      | This discrete block computes the mean value of the input signal (port In) over a running window of one cycle of a specified frequency (port Freq).
      |
      | For the first cycle of simulation (specified by the parameter "Initial frequency"), the output is held to the value of the  "Initial input" parameter.
      |
      | The value of the parameter "Minimum frequency" is used to determine the buffer size of the "Variable Transport Delay" block found inside this subsystem.
      mask init:
      | MaxDelay=1/Fmin+Ts;
      | power_initmask();
      settings: OpenFcn=power_openblockproxy();
  Discrete Variable Frequency Mean value2 : Subsystem  mask(Discrete Variable-Frequency Mean Value){Finit=Finit, Fmin=Fmin, Vinit=Real_Init, Ts=Ts}
      mask prompts: Finit "Initial frequency (Hz):"; Fmin "Minimum frequency (Hz):"; Vinit "Initial input (DC component):"; Ts "Sample time:"
      mask help:
      | This discrete block computes the mean value of the input signal (port In) over a running window of one cycle of a specified frequency (port Freq).
      |
      | For the first cycle of simulation (specified by the parameter "Initial frequency"), the output is held to the value of the  "Initial input" parameter.
      |
      | The value of the parameter "Minimum frequency" is used to determine the buffer size of the "Variable Transport Delay" block found inside this subsystem.
      mask init:
      | MaxDelay=1/Fmin+Ts;
      | power_initmask();
      settings: OpenFcn=power_openblockproxy();
  Rad->Deg. : Gain  Gain=180/pi  SaturateOnIntegerOverflow=on  OutDataTypeStr=Inherit: Same as input  ParamDataTypeStr=Inherit: Same as input
  Terminator : Terminator
  abc to dq0 : powerlib_meascontrol/Transformations/abc to dq0  Alignment=90 degrees behind phase A axis
      settings: SourceProductBaseCode=MT,PS
  Mag : Outport  VectorParamsAs1DForOutWhenUnconnected=off
  Phase : Outport  Port=2  VectorParamsAs1DForOutWhenUnconnected=off
  wires:
  w/1 -> abc to dq0/2
  Freq/1 -> Discrete Variable Frequency Mean value2/1(Freq), Discrete Variable Frequency Mean value1/1(Freq)
  Discrete Variable Frequency Mean value2/1(Mean) -> Cartesian to Polar/1  "Real"
  Rad->Deg./1 -> Phase/1
  Discrete Variable Frequency Mean value1/1(Mean) -> Cartesian to Polar/2  "Real"
  Demux/2 -> Discrete Variable Frequency Mean value1/2(In)
  Demux/1 -> Discrete Variable Frequency Mean value2/2(In)
  abc/1 -> abc to dq0/1
  abc to dq0/1 -> Demux/1
  Demux/3 -> Terminator/1
  Cartesian to Polar/1 -> Mag/1
  Cartesian to Polar/2 -> Rad->Deg./1

== system Microgrid_transition_model_FORFIG/Wind Turbine Type 4/Control/Measurement and Transformation/Discrete 3-phase PLL-Driven Positive-Sequence Active & Reactive Power/Discrete 3-phase PLL-Driven Positive-Sequence Fundamental Value2 ==
  note: Discrete 3-phase PLL-Driven Positive-Sequence Fundamental Value
  note: Pierre Giroux, Gilbert Sybille
      | Power System Simulation Laboratory
      | IREQ, Hydro-Quebc
  Freq : Inport
  w : Inport  Port=2  PortDimensions=1
  abc : Inport  Port=3  PortDimensions=3
  Cartesian to Polar : simulink_extras/Transformations/Cartesian to Polar
  Demux : Demux  Outputs=3
      settings: DisplayOption=none
  Discrete Variable Frequency Mean value1 : Subsystem  mask(Discrete Variable-Frequency Mean Value){Finit=Finit, Fmin=Fmin, Vinit=Imag_Init, Ts=Ts}
      mask prompts: Finit "Initial frequency (Hz):"; Fmin "Minimum frequency (Hz):"; Vinit "Initial input (DC component):"; Ts "Sample time:"
      mask help:
      | This discrete block computes the mean value of the input signal (port In) over a running window of one cycle of a specified frequency (port Freq).
      |
      | For the first cycle of simulation (specified by the parameter "Initial frequency"), the output is held to the value of the  "Initial input" parameter.
      |
      | The value of the parameter "Minimum frequency" is used to determine the buffer size of the "Variable Transport Delay" block found inside this subsystem.
      mask init:
      | MaxDelay=1/Fmin+Ts;
      | power_initmask();
      settings: OpenFcn=power_openblockproxy();
  Discrete Variable Frequency Mean value2 : Subsystem  mask(Discrete Variable-Frequency Mean Value){Finit=Finit, Fmin=Fmin, Vinit=Real_Init, Ts=Ts}
      mask prompts: Finit "Initial frequency (Hz):"; Fmin "Minimum frequency (Hz):"; Vinit "Initial input (DC component):"; Ts "Sample time:"
      mask help:
      | This discrete block computes the mean value of the input signal (port In) over a running window of one cycle of a specified frequency (port Freq).
      |
      | For the first cycle of simulation (specified by the parameter "Initial frequency"), the output is held to the value of the  "Initial input" parameter.
      |
      | The value of the parameter "Minimum frequency" is used to determine the buffer size of the "Variable Transport Delay" block found inside this subsystem.
      mask init:
      | MaxDelay=1/Fmin+Ts;
      | power_initmask();
      settings: OpenFcn=power_openblockproxy();
  Rad->Deg. : Gain  Gain=180/pi  SaturateOnIntegerOverflow=on  OutDataTypeStr=Inherit: Same as input  ParamDataTypeStr=Inherit: Same as input
  Terminator : Terminator
  abc to dq0 : powerlib_meascontrol/Transformations/abc to dq0  Alignment=90 degrees behind phase A axis
      settings: SourceProductBaseCode=MT,PS
  Mag : Outport  VectorParamsAs1DForOutWhenUnconnected=off
  Phase : Outport  Port=2  VectorParamsAs1DForOutWhenUnconnected=off
  wires:
  Cartesian to Polar/2 -> Rad->Deg./1
  Cartesian to Polar/1 -> Mag/1
  Demux/3 -> Terminator/1
  abc to dq0/1 -> Demux/1
  abc/1 -> abc to dq0/1
  Demux/1 -> Discrete Variable Frequency Mean value2/2(In)
  Demux/2 -> Discrete Variable Frequency Mean value1/2(In)
  Discrete Variable Frequency Mean value1/1(Mean) -> Cartesian to Polar/2  "Real"
  Rad->Deg./1 -> Phase/1
  Discrete Variable Frequency Mean value2/1(Mean) -> Cartesian to Polar/1  "Real"
  Freq/1 -> Discrete Variable Frequency Mean value1/1(Freq), Discrete Variable Frequency Mean value2/1(Freq)
  w/1 -> abc to dq0/2

== system Microgrid_transition_model_FORFIG/Wind Turbine Type 4/Control/Measurement and Transformation/Extract References/Extract References ==
  v_abc : Inport
  Add : Sum
  Constant : Constant  Value=2*pi
  Demux : Demux  Outputs=3
  Demux1 : Demux  Outputs=3
  Math Function : Math  Operator=magnitude^2  SignedPower=on  SaturateOnIntegerOverflow=on
  Math Function1 : Math  Operator=magnitude^2  SignedPower=on  SaturateOnIntegerOverflow=on
  Math Function2 : Math  Operator=mod  SignedPower=on  SaturateOnIntegerOverflow=on
  Mean (Variable Frequency) d : powerlib_meascontrol/Measurements/Mean (Variable Frequency)  Finit=f_rated  Fmin=0.9*f_rated  Vinit=0  Ts=Ts
      settings: SourceProductBaseCode=PS
  Mean (Variable Frequency) q : powerlib_meascontrol/Measurements/Mean (Variable Frequency)  Finit=f_rated  Fmin=0.9*f_rated  Vinit=0  Ts=Ts
      settings: SourceProductBaseCode=PS
  PLL : Subsystem
  Sequence Analyzer : powerlib_meascontrol/Measurements/Sequence Analyzer  Freq=f_rated  n=1  seq=Positive Negative Zero  InInit=[1, 0]  Ts=Ts
      settings: SourceProductBaseCode=PS
  Sqrt : Sqrt  SaturateOnIntegerOverflow=on
  Terminator{,1..3} (4 alike) : Terminator
  abc to dq0 : powerlib_meascontrol/Transformations/abc to dq0  Alignment=90 degrees behind phase A axis
  "rad/s -> Hz" : Gain  Gain=1/(2*pi)
  to pu : Gain  Gain=1/(sqrt(2/3)*U_rated)
  u_ref : Outport
  wt_ref : Outport  Port=2
  w_ref : Outport  Port=3
  u_frt_pu : Outport  Port=4
  wires:
  abc to dq0/1 -> Demux/1
  Demux/3 -> Terminator/1
  Math Function/1 -> Add/1
  PLL/1(angle_ref) -> abc to dq0/2, Math Function2/1
  Math Function1/1 -> Add/2
  Add/1 -> Sqrt/1
  Sqrt/1 -> u_ref/1
  v_abc/1 -> PLL/1(v_abc), to pu/1, abc to dq0/1
  Sequence Analyzer/1 -> Demux1/1
  Demux1/2 -> Terminator1/1
  Demux1/3 -> Terminator2/1
  Sequence Analyzer/2 -> Terminator3/1
  Demux1/1 -> u_frt_pu/1
  [freq] -> Mean (Variable Frequency) q/1, Mean (Variable Frequency) d/1
  Mean (Variable Frequency) d/1 -> Math Function/1
  Demux/1 -> Mean (Variable Frequency) d/2
  Mean (Variable Frequency) q/1 -> Math Function1/1
  Demux/2 -> Mean (Variable Frequency) q/2
  Constant/1 -> Math Function2/2
  Math Function2/1 -> wt_ref/1
  PLL/2(w_meas) -> w_ref/1, "rad/s -> Hz"/1
  "rad/s -> Hz"/1 -> [freq]
  to pu/1 -> Sequence Analyzer/1

== system Microgrid_transition_model_FORFIG/Wind Turbine Type 4/Control/Measurement and Transformation/Extract References/Voltage and Frequency Protection ==
  Vpos : Inport
  fgrid : Inport  Port=2
  0 ... 1 u_min : Saturate  UpperLimit=1  LowerLimit=0
  0 ... 1 u_min1 : Saturate  UpperLimit=1  LowerLimit=0
  0 ... 1 umax : Saturate  UpperLimit=1  LowerLimit=0
  0 ... 1 umax1 : Saturate  UpperLimit=1  LowerLimit=0
  Compare To Constant1 : simulink/Logic and Bit Operations/Compare To Constant  relop=>  const=fmax_delay  OutDataTypeStr=boolean
  Compare To Constant2 : simulink/Logic and Bit Operations/Compare To Constant  relop=>  const=umax_delay  OutDataTypeStr=boolean
  Compare To Constant3 : simulink/Logic and Bit Operations/Compare To Constant  relop=>  const=umin_delay  OutDataTypeStr=boolean
  Compare To Constant4 : simulink/Logic and Bit Operations/Compare To Constant  relop=>  const=fmin_delay  OutDataTypeStr=boolean
  Constant : Constant
  Counter AST fmax : Subsystem
  Counter AST fmin : Subsystem
  Counter AST umax : Subsystem
  Counter AST umin : Subsystem
  Data Type Conversion{,1..3} (4 alike) : DataTypeConversion
  Digital Clock : DigitalClock  SampleTime=Ts
  Discrete-Time Integrator{1..4} (4 alike) : DiscreteIntegrator  ExternalReset=falling  SampleTime=Ts  ICPrevOutput=DiscIntNeverNeededParam  ICPrevScaledInput=DiscIntNeverNeededParam
  Hz to pu : Gain  Gain=inv(f_rated)
  Scope : Scope  NumInputPorts=2
  Scope1 : Scope  NumInputPorts=2
  Scope2 : Scope  NumInputPorts=3
  Scope3 : Scope  NumInputPorts=3
  Scope4 : Scope  NumInputPorts=4
  V to pu : Gain  Gain=1/(sqrt(2/3)*U_rated)
  f_protection condition : Logic  Operator=OR  AllPortsSameDT=off  OutDataTypeStr=boolean
  fmax : simulink/Logic and Bit Operations/Compare To Constant  relop=>  const=fmax_protection  OutDataTypeStr=boolean
  fmin : simulink/Logic and Bit Operations/Compare To Constant  relop=<  const=fmin_protection  OutDataTypeStr=boolean
  initialize f : Switch  Criteria=u2 > Threshold  Threshold=0.5
  initialize u : Switch  Criteria=u2 > Threshold  Threshold=0.5
  protection condition : Logic  Operator=OR  AllPortsSameDT=off  OutDataTypeStr=boolean
  u_protection condition : Logic  Operator=OR  AllPortsSameDT=off  OutDataTypeStr=boolean
  umax : simulink/Logic and Bit Operations/Compare To Constant  relop=>  const=umax_protection  OutDataTypeStr=boolean
  umin : simulink/Logic and Bit Operations/Compare To Constant  relop=<  const=umin_protection  OutDataTypeStr=boolean
  u_f_protect : Outport
  wires:
  Discrete-Time Integrator1/1 -> Scope4/4, Compare To Constant1/1
  Counter AST fmin/1(Count) -> Scope2/2, 0 ... 1 u_min1/1
  Compare To Constant4/1 -> Scope2/1, Counter AST fmin/Trigger
  umax/1 -> Data Type Conversion/1
  0 ... 1 u_min/1 -> u_protection condition/2
  Discrete-Time Integrator3/1 -> Compare To Constant3/1
  Compare To Constant1/1 -> Scope3/1, Counter AST fmax/Trigger
  Counter AST umin/1(Count) -> 0 ... 1 u_min/1
  fmin/1 -> Data Type Conversion3/1
  0 ... 1 umax1/1 -> f_protection condition/1, Scope3/3
  Discrete-Time Integrator4/1 -> Compare To Constant4/1
  Counter AST fmax/1(Count) -> Scope3/2, 0 ... 1 umax1/1
  Data Type Conversion/1 -> Discrete-Time Integrator2/2, Discrete-Time Integrator2/1
  umin/1 -> Data Type Conversion1/1
  Compare To Constant3/1 -> Counter AST umin/Trigger
  Compare To Constant2/1 -> Counter AST umax/Trigger
  fmax/1 -> Scope4/2, Data Type Conversion2/1
  0 ... 1 u_min1/1 -> Scope2/3, f_protection condition/2
  Data Type Conversion3/1 -> Discrete-Time Integrator4/2, Discrete-Time Integrator4/1
  Data Type Conversion2/1 -> Scope4/3, Discrete-Time Integrator1/1, Discrete-Time Integrator1/2
  Discrete-Time Integrator2/1 -> Compare To Constant2/1
  0 ... 1 umax/1 -> u_protection condition/1
  Counter AST umax/1(Count) -> 0 ... 1 umax/1
  Data Type Conversion1/1 -> Discrete-Time Integrator3/1, Discrete-Time Integrator3/2
  fgrid/1 -> Hz to pu/1
  V to pu/1 -> initialize u/1
  Hz to pu/1 -> initialize f/1
  f_protection condition/1 -> Scope1/2, protection condition/2
  protection condition/1 -> u_f_protect/1
  Digital Clock/1 -> initialize u/2, initialize f/2
  Constant/1 -> initialize f/3, initialize u/3
  initialize u/1 -> Scope/1, umin/1, umax/1
  Vpos/1 -> V to pu/1
  u_protection condition/1 -> Scope1/1, protection condition/1
  initialize f/1 -> Scope/2, Scope4/1, fmax/1, fmin/1
